simulink model "DC_motor_LQRi_c"  (R2015b)
settings: Solver=VariableStepAuto  StartTime=0.0  StopTime=10  MaxStep=1e-2  RelTol=1e-3
settings Model: Creator=mgreiff  LastModifiedBy=mgreiff
settings DebuggingCC: AlgebraicLoopMsg=none

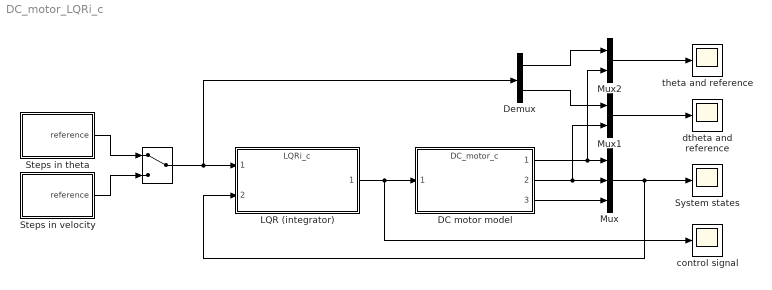
== system DC_motor_LQRi_c ==
  "    " : ManualSwitch
  DC motor model : ModelReference  ModelNameDialog=DC_motor_c.slx  SimulationMode=Normal  ModelReferenceVersion=1.7  CopyOfModelName=DC_motor_c.slx
  Demux : Demux  Outputs=2
  LQR (integrator) : ModelReference  ModelNameDialog=LQRi_c.slx  SimulationMode=Normal  ModelReferenceVersion=1.9  CopyOfModelName=LQRi_c.slx
  Mux : Mux  Inputs=3
  Mux1 : Mux  Inputs=2
  Mux2 : Mux  Inputs=2
  Steps in theta : Subsystem
  Steps in velocity : Subsystem
  System states : Scope
  control signal : Scope
  dtheta and reference : Scope
  theta and reference : Scope
  wires:
  DC motor model/1 -> Mux2/2, Mux/1
  DC motor model/2 -> Mux1/2, Mux/2
  DC motor model/3 -> Mux/3
  Mux/1 -> LQR (integrator)/2, System states/1
  Mux1/1 -> dtheta and reference/1
  LQR (integrator)/1 -> DC motor model/1, control signal/1
  Steps in theta/1(reference) -> "    "/1
  Steps in velocity/1(reference) -> "    "/2
  "    "/1 -> LQR (integrator)/1, Demux/1
  Mux2/1 -> theta and reference/1
  Demux/2 -> Mux1/1
  Demux/1 -> Mux2/1

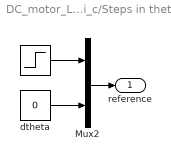
== system DC_motor_LQRi_c/Steps in theta ==
  "  " : Step  Time=0  SampleTime=0
  Mux2 : Mux  Inputs=2
  dtheta : Constant  Value=0
  reference : Outport
  wires:
  "  "/1 -> Mux2/1
  Mux2/1 -> reference/1
  dtheta/1 -> Mux2/2

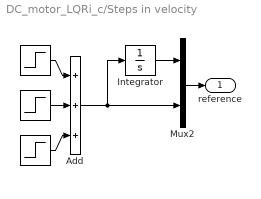
== system DC_motor_LQRi_c/Steps in velocity ==
  "  " : Step  Time=0  SampleTime=0
  "   " : Step  Time=4  After=-2  SampleTime=0
  "    " : Step  Time=8  SampleTime=0
  Add : Sum  Inputs=+++
  Integrator : Integrator
  Mux2 : Mux  Inputs=2
  reference : Outport
  wires:
  Integrator/1 -> Mux2/1
  Add/1 -> Integrator/1, Mux2/2
  Mux2/1 -> reference/1
  "   "/1 -> Add/2
  "    "/1 -> Add/3
  "  "/1 -> Add/1
